simulink model "tetherDragForce_th"  (R2018b)
settings: Solver=VariableStepAuto  StartTime=0.0  StopTime=0  RelTol=1e-3
values from neighbouring files (symbols this model uses):
  flow = [1 0 0]'    [tetherDragForce_ts.m]
  Ri_o = [R1_o Ri_o Rn_o]    [tetherDragForce_ts.m]
  Vi_o = zeros(size(Ri_o))    [tetherDragForce_ts.m]
libraries: tetherDragForce_ul x1
settings Model: Creator=asiddiq2  LastModifiedBy=asiddiq2

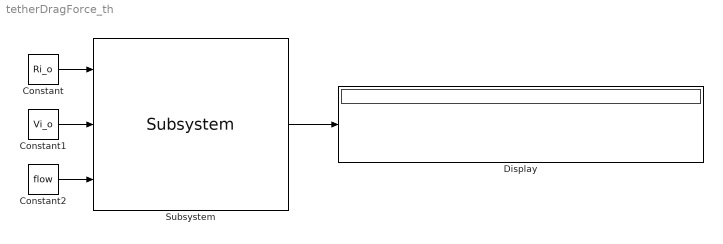
== system tetherDragForce_th ==
  Constant : Constant  Value=Ri_o
  Constant1 : Constant  Value=Vi_o
  Constant2 : Constant  Value=flow
  Display : Display
  Subsystem : tetherDragForce_ul/Subsystem  Cd=Cd  rho_fluid=rho_fluid  dia_t=dia_t
  wires:
  Constant/1 -> Subsystem/1
  Constant1/1 -> Subsystem/2
  Constant2/1 -> Subsystem/3
  Subsystem/1 -> Display/1
